simulink model "Sim2"  (R2020a)
settings: Solver=VariableStepAuto  StartTime=0.0  StopTime=0.05  RelTol=1e-6
values from neighbouring files (symbols this model uses):
  Kf = (R12+R8)/(R5+R8)    (= 1.32450331126)    [Main.m]
  Kg = 2*Km*Ubat    (= 48)    [Main.m]
  Tau1 = ((R8*R5)/(R8+R5))*C2    (= 7.43046357616e-05)    [Main.m]
  Tau2 = R21*C7    (= 4.84e-06)    [Main.m]
  tauc2 = 0.00268    [Main.m]
  Taum = Lm/Rm    (= 0.002)    [Main.m]
  Te = 200*10^(-6)    (= 0.0002)    [Main.m]
settings Model: Creator=belafki  LastModifiedBy=belafki

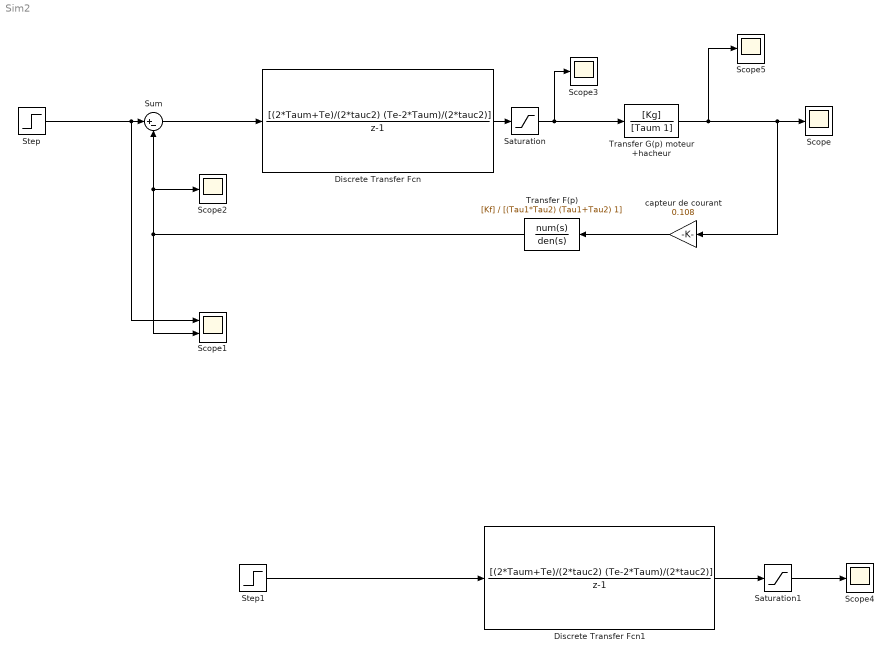
== system Sim2 ==
  Discrete Transfer Fcn : DiscreteTransferFcn  Numerator=[(2*Taum+Te)/(2*tauc2) (Te-2*Taum)/(2*tauc2)]  Denominator=[1 -1]  SampleTime=Te
  Discrete Transfer Fcn1 : DiscreteTransferFcn  Numerator=[(2*Taum+Te)/(2*tauc2) (Te-2*Taum)/(2*tauc2)]  Denominator=[1 -1]  SampleTime=Te
  Saturation : Saturate
  Saturation1 : Saturate  UpperLimit=1  LowerLimit=0
  Scope{,2..5} (5 alike) : Scope
  Scope1 : Scope  NumInputPorts=2
  Step : Step  Time=0.001  After=1.65  SampleTime=0
  Step1 : Step  Time=0.001  After=0.1  SampleTime=0
  Sum : Sum  Inputs=|+-
  Transfer F(p) : TransferFcn  Numerator=[Kf]  Denominator=[(Tau1*Tau2) (Tau1+Tau2) 1]
  Transfer G(p) moteur +hacheur : TransferFcn  Numerator=[Kg]  Denominator=[Taum 1]
  capteur de courant : Gain  Gain=0.108
  wires:
  capteur de courant/1 -> Transfer F(p)/1
  Step/1 -> Scope1/1, Sum/1
  Transfer G(p) moteur +hacheur/1 -> Scope5/1, capteur de courant/1, Scope/1
  Sum/1 -> Discrete Transfer Fcn/1
  Discrete Transfer Fcn/1 -> Saturation/1
  Transfer F(p)/1 -> Scope1/2, Scope2/1, Sum/2
  Saturation/1 -> Scope3/1, Transfer G(p) moteur +hacheur/1
  Step1/1 -> Discrete Transfer Fcn1/1
  Discrete Transfer Fcn1/1 -> Saturation1/1
  Saturation1/1 -> Scope4/1
